simulink model "pmsm_electrical_id_waveform_model"  (R2023b)
settings: Solver=FixedStepDiscrete  StartTime=0.0  StopTime=0.45  FixedStep=5e-5  RelTol=1e-3
model workspace (MAT data in the model file):
  angle_delta = [0 0.0001 0.0002 0.0003 0.0004 0.0005 0.0006 0.0007 0.0008 0.0009 0.001 0.0011 ... (8000 elements, 4000x2)]
  angle_encoder = [0 0.0001 0.0002 0.0003 0.0004 0.0005 0.0006 0.0007 0.0008 0.0009 0.001 0.0011 ... (8000 elements, 4000x2)]
  angle_residual = [0 0.0001 0.0002 0.0003 0.0004 0.0005 0.0006 0.0007 0.0008 0.0009 0.001 0.0011 ... (8000 elements, 4000x2)]
  angle_sensorless = [0 0.0001 0.0002 0.0003 0.0004 0.0005 0.0006 0.0007 0.0008 0.0009 0.001 0.0011 ... (8000 elements, 4000x2)]
  angle_true = [0 0.0001 0.0002 0.0003 0.0004 0.0005 0.0006 0.0007 0.0008 0.0009 0.001 0.0011 ... (8000 elements, 4000x2)]
  flux_id = [0 0.001 0.002 0.003 0.004 0.005 0.006 0.007 0.008 0.009 0.01 0.011 ... (2000 elements, 1000x2)]
  flux_iq = [0 0.001 0.002 0.003 0.004 0.005 0.006 0.007 0.008 0.009 0.01 0.011 ... (2000 elements, 1000x2)]
  flux_psi_est = [0 0.001 0.002 0.003 0.004 0.005 0.006 0.007 0.008 0.009 0.01 0.011 ... (2000 elements, 1000x2)]
  flux_vq = [0 0.001 0.002 0.003 0.004 0.005 0.006 0.007 0.008 0.009 0.01 0.011 ... (2000 elements, 1000x2)]
  flux_we = [0 0.001 0.002 0.003 0.004 0.005 0.006 0.007 0.008 0.009 0.01 0.011 ... (2000 elements, 1000x2)]
  step_d_current = [0 5e-05 0.0001 0.00015 0.0002 0.00025 0.0003 0.00035 0.0004 0.00045 0.0005 0.00055 ... (2002 elements, 1001x2)]
  step_d_voltage = [0 5e-05 0.0001 0.00015 0.0002 0.00025 0.0003 0.00035 0.0004 0.00045 0.0005 0.00055 ... (2002 elements, 1001x2)]
  step_q_current = [0 5e-05 0.0001 0.00015 0.0002 0.00025 0.0003 0.00035 0.0004 0.00045 0.0005 0.00055 ... (2002 elements, 1001x2)]
  step_q_voltage = [0 5e-05 0.0001 0.00015 0.0002 0.00025 0.0003 0.00035 0.0004 0.00045 0.0005 0.00055 ... (2002 elements, 1001x2)]
(part 1 of 2)
settings Model: Creator=user  LastModifiedBy=user
settings DataIOCC: SaveOutput=off

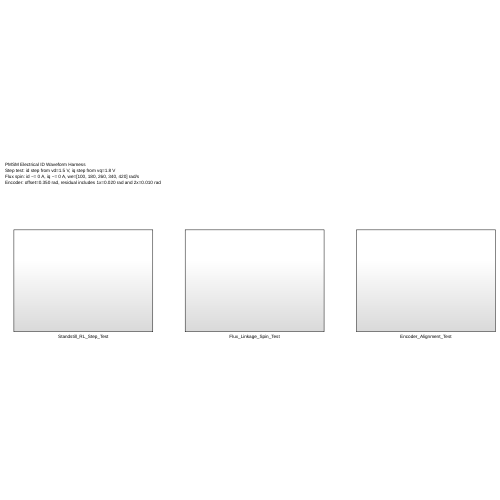
[thumbnail: Simulink's stored preview of the top-level diagram]
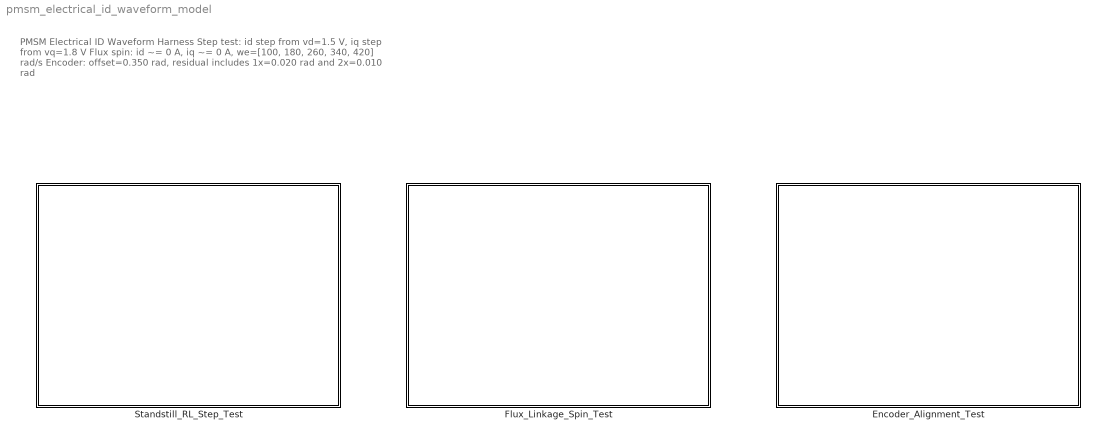
== system pmsm_electrical_id_waveform_model ==
  note: PMSM Electrical ID Waveform Harness
      | Step test: id step from vd=1.5 V, iq step from vq=1.8 V
      | Flux spin: id ~= 0 A, iq ~= 0 A, we=[100, 180, 260, 340, 420] rad/s
      | Encoder: offset=0.350 rad, residual includes 1x=0.020 rad and 2x=0.010 rad
  Encoder_Alignment_Test : Subsystem
  Flux_Linkage_Spin_Test : Subsystem
  Standstill_RL_Step_Test : Subsystem
